simulink model "FixedWing_Dynamic_Model_SIL_simulink"  (R2023a)
settings: Solver=ode4  StartTime=0.0  StopTime=timestop  FixedStep=0.004  RelTol=1e-3
model workspace (MAT data in the model file):
  sample_time = 0.004
values from neighbouring files (symbols this model uses):
  env = struct    [InitEnvironment.m]    (also in resultados_autotuning.mat = )
  F_lat = 1    [autotuning.m]    (also in resultados_autotuning.mat)
  F_lon = 1    [autotuning.m]    (also in resultados_autotuning.mat)
  frecuency = 0.012    [resultados_autotuning.mat]
  g = 9.81    [resultados_autotuning.mat]
  home_alt = 171    [InitSimulinkPlantVars.m]    (also in resultados_autotuning.mat)
  home_lat = 39.49738807491014    (= 39.4973880749)    [InitSimulinkPlantVars.m]    (also in resultados_autotuning.mat)
  home_lon = -0.6268122488722822    (= -0.626812248872)    [InitSimulinkPlantVars.m]    (also in resultados_autotuning.mat)
  LC =     [resultados_autotuning.mat]
  mission =     [resultados_autotuning.mat]
  nav = 0    [autotuning.m]    (also in resultados_autotuning.mat)
  nwap = 9    [resultados_autotuning.mat]
  pitch_D = p(3)    [Error_Medio_Cuadratico_lon.m]    (also in autotuning.m = gaDat3.xmin(8); resultados_autotuning.mat = 0.0221525560229)
  pitch_ff = p(5)    [Error_Medio_Cuadratico_lon.m]    (also in autotuning.m = gaDat3.xmin(10); resultados_autotuning.mat = 1.57455388381)
  pitch_I = p(2)    [Error_Medio_Cuadratico_lon.m]    (also in autotuning.m = gaDat3.xmin(7); resultados_autotuning.mat = 4.90608990643)
  pitch_P = p(1)    [Error_Medio_Cuadratico_lon.m]    (also in autotuning.m = gaDat3.xmin(6); resultados_autotuning.mat = 2.28969592616)
  poswp = [0 203.689232032 39.9384744604 259.790159417 479.641844374 368.12834454 131.944883572 -98.7095328994 459.946011169 0 253.211382055 414.656010519 ... (27 elements, 9x3)]    [resultados_autotuning.mat]
  roll_D = gaDat3.xmin(3)    [autotuning.m]    (also in resultados_autotuning.mat = 0.180903871459)
  roll_ff = gaDat3.xmin(5)    [autotuning.m]    (also in resultados_autotuning.mat = 2.84810617708)
  roll_I = gaDat3.xmin(2)    [autotuning.m]    (also in resultados_autotuning.mat = 3.06744673684)
  roll_P = gaDat3.xmin(1)    [autotuning.m]    (also in resultados_autotuning.mat = 5.38476214824)
  tc_pitch = p(4)    [Error_Medio_Cuadratico_lon.m]    (also in autotuning.m = gaDat3.xmin(9); resultados_autotuning.mat = 0.664298153877)
  tc_roll = gaDat3.xmin(4)    [autotuning.m]    (also in resultados_autotuning.mat = 0.655996177908)
  TEBCL =     [resultados_autotuning.mat]
  TECL =     [resultados_autotuning.mat]
  TECS =     [resultados_autotuning.mat]
  throttle_sp = 0.6    [autotuning.m]    (also in resultados_autotuning.mat)
  uavData = struct    [InitFixedWingParam.m]    (also in resultados_autotuning.mat = )
  V_cruise = [15 15 15 20 25 25 20 15 15]    [resultados_autotuning.mat]
  yaw_D = gaDat3.xmin(13)    [autotuning.m]    (also in resultados_autotuning.mat = 0.0051969904619)
  yaw_ff = gaDat3.xmin(14)    [autotuning.m]    (also in resultados_autotuning.mat = 1.81739785006)
  yaw_I = gaDat3.xmin(12)    [autotuning.m]    (also in resultados_autotuning.mat = 7.2697636977)
  yaw_P = gaDat3.xmin(11)    [autotuning.m]    (also in resultados_autotuning.mat = 2.788657103)
undefined symbols (not defined in the file or in its folder): DiscIntNeverNeededParam, Earth, WGS84
libraries: aerolibactuator x5, aerolibasang x4, slpidlib x3, uavalgslib x2, aerolibatmos2 x2, shared6dof x1, aerolibtransform2 x1, aerolibconvert2 x1, simulink_extras x1
(part 3 of 3)

== system FixedWing_Dynamic_Model_SIL_simulink/Dynamics/Fixed-wing UAV Dynamics/Force and Moment Calculation/Aerodynamic Forces and Moments/Compute Body Frame Forces and Moments/Wind frame F& M/Longitudinal Channel/CL ==
  alpha : Inport
  alpha_dot : Inport  Port=2
  dE : Inport  Port=3
  dF : Inport  Port=4
  p,q,r : Inport  Port=5
  Airspeed : Inport  Port=6
  CL0 : Constant  Value=uavData.aero.CL0
      settings: AttributesFormatString=%<Value>
  CLDe : Constant  Value=uavData.aero.CLDe
      settings: AttributesFormatString=%<Value>
  CLa : Constant  Value=uavData.aero.CLa
      settings: AttributesFormatString=%<Value>
  CLa_dot : Constant  Value=uavData.aero.CLa_dot
      settings: AttributesFormatString=%<Value>
  CmDe1 : Constant  Value=uavData.aero.CLDf
      settings: AttributesFormatString=%<Value>
  Lift due to pitch rate : Subsystem
  Product{1..2,4..5} (4 alike) : Product  SaturateOnIntegerOverflow=on  OutDataTypeStr=Inherit: Same as first input
  Sum : Sum  Inputs=++++++  SaturateOnIntegerOverflow=on
  CL : Outport  VectorParamsAs1DForOutWhenUnconnected=off
  wires:
  CL0/1 -> Sum/1
  Airspeed/1 -> Lift due to pitch rate/2(Airspeed)
  p,q,r/1 -> Lift due to pitch rate/1(p,q,r)
  Lift due to pitch rate/1(CLq) -> Sum/6
  Product2/1 -> Sum/5
  Product1/1 -> Sum/4
  Product5/1 -> Sum/3
  CmDe1/1 -> Product2/1
  dF/1 -> Product2/2
  Sum/1 -> CL/1
  dE/1 -> Product1/2
  CLDe/1 -> Product1/1
  alpha_dot/1 -> Product5/2
  CLa_dot/1 -> Product5/1
  alpha/1 -> Product4/2
  CLa/1 -> Product4/1
  Product4/1 -> Sum/2

== system FixedWing_Dynamic_Model_SIL_simulink/Dynamics/Fixed-wing UAV Dynamics/Force and Moment Calculation/Aerodynamic Forces and Moments/Compute Body Frame Forces and Moments/Wind frame F& M/Longitudinal Channel/Cm ==
  alpha : Inport
  De : Inport  Port=2
  Df : Inport  Port=3
  p,q,r : Inport  Port=4
  Cm0 : Constant  Value=uavData.aero.Cm0
      settings: AttributesFormatString=%<Value>
  CmDe : Constant  Value=uavData.aero.CmDe
      settings: AttributesFormatString=%<Value>
  CmDf : Constant  Value=uavData.aero.CmDf
      settings: AttributesFormatString=%<Value>
  Cma : Constant  Value=uavData.aero.Cma
      settings: AttributesFormatString=%<Value>
  Cma1 : Constant  Value=uavData.aero.Cmq
      settings: AttributesFormatString=%<Value>
  Get q : Selector  InputPortWidth=3  IndexOptions=Index vector (dialog)  Indices=2  OutputSizes=[(-2)]
  Product1 : Product  Inputs=***/  SaturateOnIntegerOverflow=on  OutDataTypeStr=Inherit: Same as first input
  Product2 : Product  SaturateOnIntegerOverflow=on  OutDataTypeStr=Inherit: Same as first input
  Product3 : Product  SaturateOnIntegerOverflow=on  OutDataTypeStr=Inherit: Same as first input
  Product4 : Product  SaturateOnIntegerOverflow=on  OutDataTypeStr=Inherit: Same as first input
  Sum : Sum  Inputs=+++++  SaturateOnIntegerOverflow=on
  chord : Constant  Value=uavData.geometry.chord
      settings: AttributesFormatString=%<Value>
  elarm : Constant  Value=uavData.geometry.elarm
      settings: AttributesFormatString=%<Value>
  Cm : Outport  VectorParamsAs1DForOutWhenUnconnected=off
  wires:
  chord/1 -> Product1/4
  elarm/1 -> Product1/3
  Get q/1 -> Product3/2
  Product3/1 -> Sum/5  "cmq"
  p,q,r/1 -> Get q/1
  Cma1/1 -> Product3/1
  Product1/1 -> Sum/3  "cmde"
  Product4/1 -> Sum/2  "cma"
  Sum/1 -> Cm/1  "total"
  De/1 -> Product1/2
  CmDe/1 -> Product1/1
  alpha/1 -> Product4/2
  Cma/1 -> Product4/1
  Df/1 -> Product2/2
  CmDf/1 -> Product2/1
  Product2/1 -> Sum/4  "cmdf"
  Cm0/1 -> Sum/1  "cm0"

== system FixedWing_Dynamic_Model_SIL_simulink/Dynamics/Fixed-wing UAV Dynamics/Force and Moment Calculation/Aerodynamic Forces and Moments/Compute Body Frame Forces and Moments/Wind frame F& M/Lateral Channel/Cl/roll factors ==
  p,q,r : Inport
  Airspeed : Inport  Port=2
  Constant : Constant  Value=uavData.aero.Clp
      settings: AttributesFormatString=%<Value>
  Constant1 : Constant  Value=uavData.aero.Clr
      settings: AttributesFormatString=%<Value>
  Get p : Selector  InputPortWidth=3  IndexOptions=Index vector (dialog)  Indices=1  OutputSizes=[(-2)]
  Get r : Selector  InputPortWidth=3  IndexOptions=Index vector (dialog)  Indices=3  OutputSizes=[(-2)]
  Product : Product  SaturateOnIntegerOverflow=on  OutDataTypeStr=Inherit: Same as first input
  Product1 : Product  SaturateOnIntegerOverflow=on  OutDataTypeStr=Inherit: Same as first input
  roll rate fact : Subsystem
  yaw rate fact : Subsystem
  Clp : Outport  VectorParamsAs1DForOutWhenUnconnected=off
  Clr : Outport  Port=2  VectorParamsAs1DForOutWhenUnconnected=off
  wires:
  Get r/1 -> yaw rate fact/1(r)
  p,q,r/1 -> Get r/1, Get p/1
  Get p/1 -> roll rate fact/1(p)
  Airspeed/1 -> yaw rate fact/2(Airspeed), roll rate fact/2(Airspeed)
  yaw rate fact/1(Yaw Rate Fac) -> Product1/2
  Constant1/1 -> Product1/1
  roll rate fact/1(Roll Rate Fac) -> Product/2
  Constant/1 -> Product/1
  Product1/1 -> Clr/1
  Product/1 -> Clp/1

== system FixedWing_Dynamic_Model_SIL_simulink/Dynamics/Fixed-wing UAV Dynamics/Force and Moment Calculation/Aerodynamic Forces and Moments/Compute Body Frame Forces and Moments/Wind frame F& M/Lateral Channel/Cn/yaw factors ==
  p,q,r : Inport
  Airspeed : Inport  Port=2
  Constant : Constant  Value=uavData.aero.Cnp
      settings: AttributesFormatString=%<Value>
  Constant1 : Constant  Value=uavData.aero.Cnr
      settings: AttributesFormatString=%<Value>
  Get p : Selector  InputPortWidth=3  IndexOptions=Index vector (dialog)  Indices=1  OutputSizes=[(-2)]
  Get r : Selector  InputPortWidth=3  IndexOptions=Index vector (dialog)  Indices=3  OutputSizes=[(-2)]
  Product : Product  SaturateOnIntegerOverflow=on  OutDataTypeStr=Inherit: Same as first input
  Product1 : Product  SaturateOnIntegerOverflow=on  OutDataTypeStr=Inherit: Same as first input
  roll rate fact : Subsystem
  yaw rate fact : Subsystem
  Cnp : Outport  VectorParamsAs1DForOutWhenUnconnected=off
  Cnr : Outport  Port=2  VectorParamsAs1DForOutWhenUnconnected=off
  wires:
  Airspeed/1 -> yaw rate fact/2(Airspeed), roll rate fact/2(Airspeed)
  Get r/1 -> yaw rate fact/1(r)
  p,q,r/1 -> Get r/1, Get p/1
  Get p/1 -> roll rate fact/1(p)
  roll rate fact/1(Roll Rate Fac) -> Product/2
  Constant/1 -> Product/1
  yaw rate fact/1(Yaw Rate Fac) -> Product1/2
  Constant1/1 -> Product1/1
  Product1/1 -> Cnr/1
  Product/1 -> Cnp/1

== system FixedWing_Dynamic_Model_SIL_simulink/Dynamics/Fixed-wing UAV Dynamics/Force and Moment Calculation/Aerodynamic Forces and Moments/Compute Body Frame Forces and Moments/Wind frame F& M/Longitudinal Channel/CL/Lift due to pitch rate ==
  p,q,r : Inport
  Airspeed : Inport  Port=2
  Constant : Constant  Value=uavData.aero.CLq
      settings: AttributesFormatString=%<Value>
  Get q : Selector  InputPortWidth=3  IndexOptions=Index vector (dialog)  Indices=2  OutputSizes=[(-2)]
  Product : Product  SaturateOnIntegerOverflow=on  OutDataTypeStr=Inherit: Same as first input
  pitch rate factor : Subsystem
  CLq : Outport  VectorParamsAs1DForOutWhenUnconnected=off
  wires:
  Airspeed/1 -> pitch rate factor/2(Airspeed)
  Get q/1 -> pitch rate factor/1(q)
  p,q,r/1 -> Get q/1
  Product/1 -> CLq/1
  pitch rate factor/1(Pitch Rate Fac) -> Product/2
  Constant/1 -> Product/1

== system FixedWing_Dynamic_Model_SIL_simulink/Dynamics/Fixed-wing UAV Dynamics/Force and Moment Calculation/Aerodynamic Forces and Moments/Compute Body Frame Forces and Moments/Wind frame F& M/Lateral Channel/Cl/roll factors/roll rate fact ==
  p : Inport
  Airspeed : Inport  Port=2
  Cmq1 : Constant  Value=.5
      settings: AttributesFormatString=%<Value>
  Cmq2 : Constant  Value=uavData.geometry.span
      settings: AttributesFormatString=%<Value>
  Product : Product  Inputs=***/  SaturateOnIntegerOverflow=on  OutDataTypeStr=Inherit: Same as first input
  Saturation : Saturate  UpperLimit=inf  LowerLimit=0.1
      settings: AttributesFormatString="[%<LowerLimit>  %<UpperLimit>]"
  Roll Rate Fac : Outport  VectorParamsAs1DForOutWhenUnconnected=off
  wires:
  Saturation/1 -> Product/4
  Airspeed/1 -> Saturation/1
  Cmq2/1 -> Product/3
  Cmq1/1 -> Product/2
  p/1 -> Product/1
  Product/1 -> Roll Rate Fac/1

== system FixedWing_Dynamic_Model_SIL_simulink/Dynamics/Fixed-wing UAV Dynamics/Force and Moment Calculation/Aerodynamic Forces and Moments/Compute Body Frame Forces and Moments/Wind frame F& M/Lateral Channel/Cl/roll factors/yaw rate fact ==
  r : Inport
  Airspeed : Inport  Port=2
  Cmq3 : Constant  Value=.5
      settings: AttributesFormatString=%<Value>
  Cmq4 : Constant  Value=uavData.geometry.span
      settings: AttributesFormatString=%<Value>
  Product1 : Product  Inputs=***/  SaturateOnIntegerOverflow=on  OutDataTypeStr=Inherit: Same as first input
  Saturation : Saturate  UpperLimit=inf  LowerLimit=0.1
      settings: AttributesFormatString="[%<LowerLimit>  %<UpperLimit>]"
  Yaw Rate Fac : Outport  VectorParamsAs1DForOutWhenUnconnected=off
  wires:
  Product1/1 -> Yaw Rate Fac/1
  r/1 -> Product1/1
  Cmq3/1 -> Product1/2
  Cmq4/1 -> Product1/3
  Airspeed/1 -> Saturation/1
  Saturation/1 -> Product1/4

== system FixedWing_Dynamic_Model_SIL_simulink/Dynamics/Fixed-wing UAV Dynamics/Force and Moment Calculation/Aerodynamic Forces and Moments/Compute Body Frame Forces and Moments/Wind frame F& M/Lateral Channel/Cn/yaw factors/roll rate fact ==
  p : Inport
  Airspeed : Inport  Port=2
  Cmq1 : Constant  Value=.5
      settings: AttributesFormatString=%<Value>
  Cmq2 : Constant  Value=uavData.geometry.span
      settings: AttributesFormatString=%<Value>
  Product : Product  Inputs=***/  SaturateOnIntegerOverflow=on  OutDataTypeStr=Inherit: Same as first input
  Saturation : Saturate  UpperLimit=inf  LowerLimit=0.1
      settings: AttributesFormatString="[%<LowerLimit>  %<UpperLimit>]"
  Roll Rate Fac : Outport  VectorParamsAs1DForOutWhenUnconnected=off
  wires:
  Saturation/1 -> Product/4
  Airspeed/1 -> Saturation/1
  Cmq2/1 -> Product/3
  Cmq1/1 -> Product/2
  p/1 -> Product/1
  Product/1 -> Roll Rate Fac/1

== system FixedWing_Dynamic_Model_SIL_simulink/Dynamics/Fixed-wing UAV Dynamics/Force and Moment Calculation/Aerodynamic Forces and Moments/Compute Body Frame Forces and Moments/Wind frame F& M/Lateral Channel/Cn/yaw factors/yaw rate fact ==
  r : Inport
  Airspeed : Inport  Port=2
  Cmq3 : Constant  Value=.5
      settings: AttributesFormatString=%<Value>
  Cmq4 : Constant  Value=uavData.geometry.span
      settings: AttributesFormatString=%<Value>
  Product1 : Product  Inputs=***/  SaturateOnIntegerOverflow=on  OutDataTypeStr=Inherit: Same as first input
  Saturation : Saturate  UpperLimit=inf  LowerLimit=0.1
      settings: AttributesFormatString="[%<LowerLimit>  %<UpperLimit>]"
  Yaw Rate Fac : Outport  VectorParamsAs1DForOutWhenUnconnected=off
  wires:
  Product1/1 -> Yaw Rate Fac/1
  r/1 -> Product1/1
  Cmq3/1 -> Product1/2
  Cmq4/1 -> Product1/3
  Airspeed/1 -> Saturation/1
  Saturation/1 -> Product1/4

== system FixedWing_Dynamic_Model_SIL_simulink/Dynamics/Fixed-wing UAV Dynamics/Force and Moment Calculation/Aerodynamic Forces and Moments/Compute Body Frame Forces and Moments/Wind frame F& M/Longitudinal Channel/CL/Lift due to pitch rate/pitch rate factor ==
  q : Inport
  Airspeed : Inport  Port=2
  Cmq2 : Constant  Value=uavData.geometry.chord
      settings: AttributesFormatString=%<Value>
  Product : Product  Inputs=**/  SaturateOnIntegerOverflow=on  OutDataTypeStr=Inherit: Same as first input
  Saturation : Saturate  UpperLimit=inf  LowerLimit=0.1
      settings: AttributesFormatString="[%<LowerLimit>  %<UpperLimit>]"
  Pitch Rate Fac : Outport  VectorParamsAs1DForOutWhenUnconnected=off
  wires:
  Saturation/1 -> Product/3
  Cmq2/1 -> Product/2
  Airspeed/1 -> Saturation/1
  q/1 -> Product/1
  Product/1 -> Pitch Rate Fac/1

== matlab function FixedWing_Dynamic_Model_SIL_simulink/Controllers/Total Energy control system/Total energy balance control loop/MATLAB Function1 ==
  data: SEB_rate_correction input; pitch_setpoint_1 output; V_TAS input
function pitch_setpoint_1  = seb_to_pitch(SEB_rate_correction,V_TAS)

g = 9.81;
airspeed_for_seb_rate = 15;

if V_TAS > 10^-6

airspeed_for_seb_rate = V_TAS;
end 

climb_angle_to_SEB_rate = airspeed_for_seb_rate*g;

pitch_setpoint_1 = SEB_rate_correction/climb_angle_to_SEB_rate;

== matlab function FixedWing_Dynamic_Model_SIL_simulink/Controllers/L1 Controller/MATLAB Function1 ==
  data: eta input; eta output
function eta = fcn(eta)
eta = mod(eta,2*pi);
if eta>pi
    eta = eta-2*pi;
end

== matlab function FixedWing_Dynamic_Model_SIL_simulink/Controllers/Attitude Controller/MATLAB Function2 ==
  data: roll_setpoint input; roll_body_rate_setpoint_raw output; roll input; euler_yaw_rate_setpoint input; tc input; pitch input
function roll_body_rate_setpoint_raw = roll_crtl(roll_setpoint,roll,euler_yaw_rate_setpoint,tc,pitch)
roll_error = roll_setpoint-roll;
euler_rate_setpoint = roll_error /tc;
roll_body_rate_setpoint_raw = euler_rate_setpoint - sin(pitch)*euler_yaw_rate_setpoint;

== matlab function FixedWing_Dynamic_Model_SIL_simulink/Controllers/Attitude Controller/MATLAB Function3 ==
  data: pitch_body_rate_setpoint_raw output; pitch input; euler_yaw_rate_setpoint input; roll input; euler_rate_setpoint_pitch input
function pitch_body_rate_setpoint_raw  = pitch_crtl(pitch,euler_yaw_rate_setpoint,roll,euler_rate_setpoint_pitch)

pitch_body_rate_setpoint_raw = cos(roll)*euler_rate_setpoint_pitch+cos(pitch)*sin(roll)*euler_yaw_rate_setpoint;

== matlab function FixedWing_Dynamic_Model_SIL_simulink/Controllers/Attitude Controller/MATLAB Function4 ==
  data: roll input; yaw_body_rate_setpoint_raw output; pitch input; euler_pitch_rate_setpoint input; euler_rate_setpoint_yaw input
function yaw_body_rate_setpoint_raw    = yaw_crtl(roll,pitch,euler_pitch_rate_setpoint,euler_rate_setpoint_yaw)

yaw_body_rate_setpoint_raw = -sin(roll)*euler_pitch_rate_setpoint+cos(roll)*cos(pitch)*euler_rate_setpoint_yaw;

== matlab function FixedWing_Dynamic_Model_SIL_simulink/Controllers/MATLAB Function1 ==
  data: tas_error_percentage input; ratio_undersped output; equivalent_airspeed_trim input; tas_min input; tas input
function ratio_undersped = ratio_underspeed(tas_error_percentage,equivalent_airspeed_trim,tas_min,tas)

tas_error_bound = tas_error_percentage*equivalent_airspeed_trim;
tas_undersped_soft_bound = tas_error_bound*equivalent_airspeed_trim;

tas_fully_undersped = max(tas_min-tas_error_bound-tas_undersped_soft_bound,0);
tas_starting_to_undersped = max(tas_min-tas_error_bound,tas_fully_undersped);

ratio_undersped = 1-((norm(tas)-tas_fully_undersped)/max(tas_starting_to_undersped-tas_fully_undersped,10^-6));

== matlab function FixedWing_Dynamic_Model_SIL_simulink/Controllers/Attitude Controller/MATLAB Function5 ==
  data: roll input; euler_rate_setpoint_yaw output; euler_rate_setpoint_pitch output; roll_setpoint input; pitch input; airspeed input; pitch_setpoint input; tc input
function [euler_rate_setpoint_yaw,euler_rate_setpoint_pitch] = euler_rate(roll,roll_setpoint,pitch,airspeed,pitch_setpoint,tc)
g = 9.81;
contrained_roll = min(max(roll,-abs(roll_setpoint)),abs(roll_setpoint));
euler_rate_setpoint_yaw = tan(contrained_roll)*cos(pitch)*g/airspeed; % turn coordination

pitch_error = pitch_setpoint-pitch;
euler_rate_setpoint_pitch = pitch_error/tc;

== matlab function FixedWing_Dynamic_Model_SIL_simulink/Controllers/Total Energy control system/Total energy control loop/MATLAB Function4 ==
  data: throttle_max input; throttle_min input; throttle_integ_input input; throttle_integ_state output
function throttle_integ_state = T_integ(throttle_max,throttle_min, throttle_integ_input)

if throttle_integ_input >= throttle_max
    throttle_integ_input = min(0,throttle_integ_input);
elseif throttle_integ_input<= throttle_min
    throttle_integ_input = max(0,throttle_integ_input);
end
    throttle_integ_state = throttle_integ_input;

== matlab function FixedWing_Dynamic_Model_SIL_simulink/Controllers/Total Energy control system/Total energy balance control loop/MATLAB Function4 ==
  data: vert_accel_limit input; pitch_increment output; V_TAS input
function pitch_increment = pitch_incre(vert_accel_limit,V_TAS)

pitch_increment = vert_accel_limit / max(V_TAS,10^-6);

== matlab function FixedWing_Dynamic_Model_SIL_simulink/Controllers/Total Energy control system/Total energy balance control loop/MATLAB Function5 ==
  data: pitch_setpoint input; pitch_increment input; pitch_setpoint output
function pitch_setpoint = pitch_incre_lim(pitch_setpoint,pitch_increment)
pitch_setpoint = min(max(pitch_setpoint,pitch_setpoint-pitch_increment),pitch_setpoint+pitch_increment);

== matlab function FixedWing_Dynamic_Model_SIL_simulink/Controllers/MATLAB Function4 ==
  data: ratio_undersped input; weight_spe output; pitch_speed_weight input; weight_ske output
function [weight_spe,weight_ske] = weight(ratio_undersped,pitch_speed_weight)

pitch_speed_weight = min(max(pitch_speed_weight,0),2);

if ratio_undersped>10^-6
    pitch_speed_weight = 2*ratio_undersped+(1-ratio_undersped)*pitch_speed_weight;
end

weight_spe = min(max(2-pitch_speed_weight,0),1);
weight_ske = min(max(pitch_speed_weight,0),1);

== matlab function FixedWing_Dynamic_Model_SIL_simulink/Controllers/Total Energy control system/Total energy control loop/MATLAB Function2 ==
  data: ste_rate input; ste_rate_max input; T_FF output; ste_rate_min input; throttle_max input; throttle_min input; throttle_trim input
function T_FF  = T_predicted(ste_rate,ste_rate_max, ste_rate_min, throttle_max, throttle_min, throttle_trim)
throttle_above_trim_per_ste_rate = (throttle_max - throttle_trim)/ste_rate_max;
throttle_below_trim_per_ste_rate = (throttle_trim - throttle_min)/ste_rate_min;

if ste_rate >= 10^-6
    T_FF = throttle_trim + ste_rate*throttle_above_trim_per_ste_rate;
else
    T_FF = throttle_trim - ste_rate*throttle_below_trim_per_ste_rate;
end

== matlab function FixedWing_Dynamic_Model_SIL_simulink/Controllers/Total Energy control system/Total energy balance control loop/MATLAB Function2 ==
  data: SEB_rate_correction input; pitch_setpoint_1 output; V_TAS input
function pitch_setpoint_1  = seb_to_pitch(SEB_rate_correction,V_TAS)

g = 9.81;
airspeed_for_seb_rate = 15;

if V_TAS > 10^-6

airspeed_for_seb_rate = V_TAS;
end 

climb_angle_to_SEB_rate = airspeed_for_seb_rate*g;

pitch_setpoint_1 = SEB_rate_correction/climb_angle_to_SEB_rate;

== matlab function FixedWing_Dynamic_Model_SIL_simulink/Controllers/Seguimiento waypoints/MATLAB Function4 ==
  data: Vcruise input; velocidad output; current_wp input; poswp input; nwap input
function velocidad  = vel(Vcruise, current_wp,poswp,nwap)

velocidad = Vcruise(1);
for i = 1:nwap
    if current_wp(1) == poswp(i,1)
        velocidad = Vcruise(i);
    end
end

== matlab function FixedWing_Dynamic_Model_SIL_simulink/Controllers/MATLAB Function ==
  data: vxyz input; course output; gndspeed output
function [course, gndspeed] = cour_gnds(vxyz)

vx = vxyz(1);
vy = vxyz(2);

course = atan2(vy,vx);
gndspeed = norm([vx,vy]);

== matlab function FixedWing_Dynamic_Model_SIL_simulink/Controllers/Total Energy control system/Total energy balance control loop/MATLAB Function3 ==
  data: pitch_max input; pitch_integ_state output; pitch_min input; pitch_integ_input input
function pitch_integ_state = p_integ(pitch_max,pitch_min,pitch_integ_input)
if pitch_integ_input >= pitch_max
    pitch_integ_input = min(pitch_integ_input,0);
elseif pitch_integ_input <= pitch_min
    pitch_integ_input = max(pitch_integ_input,0);
end
pitch_integ_state = pitch_integ_input;

== matlab function FixedWing_Dynamic_Model_SIL_simulink/Controllers/Seguimiento waypoints/MATLAB Function2 ==
  data: toWP input; wps output; fromWP input; alt output
function [wps, alt]= waypoints_alt(toWP, fromWP)
    wps = zeros(2,3); 
    wps = [fromWP'; toWP'];
    alt = -toWP(3);
end

== matlab function FixedWing_Dynamic_Model_SIL_simulink/Controllers/MATLAB Function2 ==
  data: max_climb_rate input; ste_rate_to_throttle output; min_sink_rate input; ste_rate_max output; ste_rate_min output
function [ste_rate_to_throttle,ste_rate_max,ste_rate_min]  = ste(max_climb_rate,min_sink_rate)
 g = 9.81;
ste_rate_max = max(max_climb_rate,10^-6)*g;
ste_rate_min = -max(min_sink_rate,10^-6)*g;

ste_rate_to_throttle = 1/(ste_rate_max-ste_rate_min);

== matlab function FixedWing_Dynamic_Model_SIL_simulink/Controllers/MATLAB Function3 ==
  data: ste_rate_max input; airspeed_rate_output output; ste_rate_min input; V_TAS input; airspeed_rate input
function airspeed_rate_output = V_rate(ste_rate_max,ste_rate_min,V_TAS,airspeed_rate)
max_tas_rate_sp = 0.5*ste_rate_max/max(V_TAS,10^-6);
min_tas_rate_sp = 0.5*ste_rate_min/max(V_TAS,10^-6);

airspeed_rate_output = min(max(airspeed_rate,min_tas_rate_sp),max_tas_rate_sp);
